simulink model "sim_actuator"  (R2024b)
settings: Solver=VariableStepAuto  StartTime=0  StopTime=1  FixedStep=dt  RelTol=1e-8
settings Model: Creator=yevge  LastModifiedBy=yevge
settings DebuggingCC: AlgebraicLoopMsg=error  CheckMatrixSingularityMsg=error

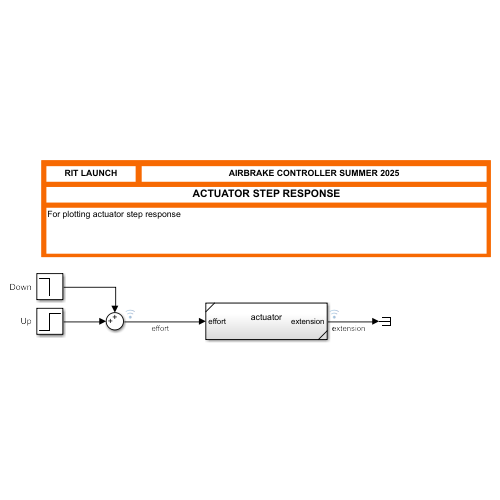
[thumbnail: Simulink's stored preview of the top-level diagram]
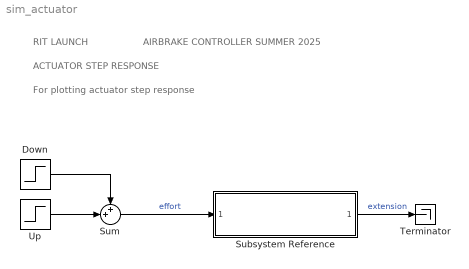
== system sim_actuator ==
  note: RIT LAUNCH
  note: For plotting actuator step response
  note: AIRBRAKE CONTROLLER SUMMER 2025
  note: ACTUATOR STEP RESPONSE
  Down : Step  Time=0.6  After=-1  SampleTime=0
  Subsystem Reference : Subsystem  ReferencedSubsystem=actuator
  Sum : Sum  Inputs=++|
  Terminator : Terminator
  Up : Step  Time=0.1  SampleTime=0
  wires:
  Up/1 -> Sum/2
  Down/1 -> Sum/1
  Sum/1 -> Subsystem Reference/1  "effort"
  Subsystem Reference/1 -> Terminator/1  "extension"
